simulink model "psbaccurrent"  (Simulink 6.0)
settings: Solver=VariableStepDiscrete  SolverMode=SingleTasking  StartTime=0.0  StopTime=0.5  MaxStep=1e-03  RelTol=1e-3  AbsTol=1e-6
libraries: powerlib2 x5
settings Model: Creator=patrice  LastModifiedBy=batserve  ExtModeTrigMode=oneshot  ExtModeArmWhenConnect=off  ExtModeAutoUpdateStatusClock=off
settings DataIOCC: LimitDataPoints=off
settings OptimizationCC: BooleanDataType=off
settings DebuggingCC: SolverPrmCheckMsg=none
settings HardwareCC: TargetUnknown=on
settings RTWCC: TemplateMakefile=grt_unix.tmf

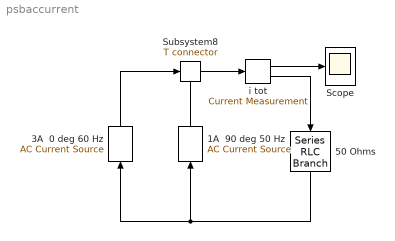
== system psbaccurrent ==
  1A  90 deg 50 Hz : powerlib2/Electrical Sources/AC Current Source  Tag=PoWeRsYsTeMbLoCk  Orientation=up  A=1  P=90  F=50  stime=0  mesure=None  PSBOutputType=1
  3A  0 deg 60 Hz : powerlib2/Electrical Sources/AC Current Source  Tag=PoWeRsYsTeMbLoCk  Orientation=up  A=3  P=0  F=60  stime=0  mesure=None  PSBOutputType=1
  "50 Ohms " : powerlib2/Elements/Series RLC Branch  Tag=PoWeRsYsTeMbLoCk  Orientation=down  a=50  b=0  c=inf  mesure=None  PSBOutputType=1
  Scope : Scope
      settings: TickLabels=on  TimeRange=0.5  DataFormat=Array
  Subsystem8 : powerlib2/Connectors/T connector  Tag=PoWeRsYsTeMbLoCk  PSBOutputType=1
  i tot : powerlib2/Measurements/Current Measurement  Tag=PoWeRsYsTeMmEaSuReMeNt  PSBOutputType=01  PSBequivalent=1
  wires:
  Subsystem8/1 -> i tot/1
  i tot/2 -> "50 Ohms "/1
  "50 Ohms "/1 -> 3A  0 deg 60 Hz/1, 1A  90 deg 50 Hz/1
  i tot/1 -> Scope/1
  3A  0 deg 60 Hz/1 -> Subsystem8/1
  1A  90 deg 50 Hz/1 -> Subsystem8/Enable
